simulink model "CAN_receiver"  (R2024a)
settings: Solver=FixedStepAuto  StartTime=0.0  StopTime=3  FixedStep=0.0025  RelTol=1e-3
undefined symbols (not defined in the file): CAN_Device, ImuSampleTime, Kvaser
libraries: sldrtlib x18
settings Model: Creator=17739  LastModifiedBy=17739
settings RTWCC: GPUComputeCapability=3.5

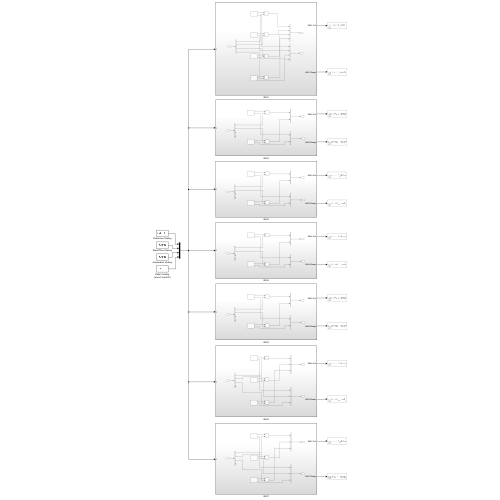
[thumbnail: Simulink's stored preview of the top-level diagram]
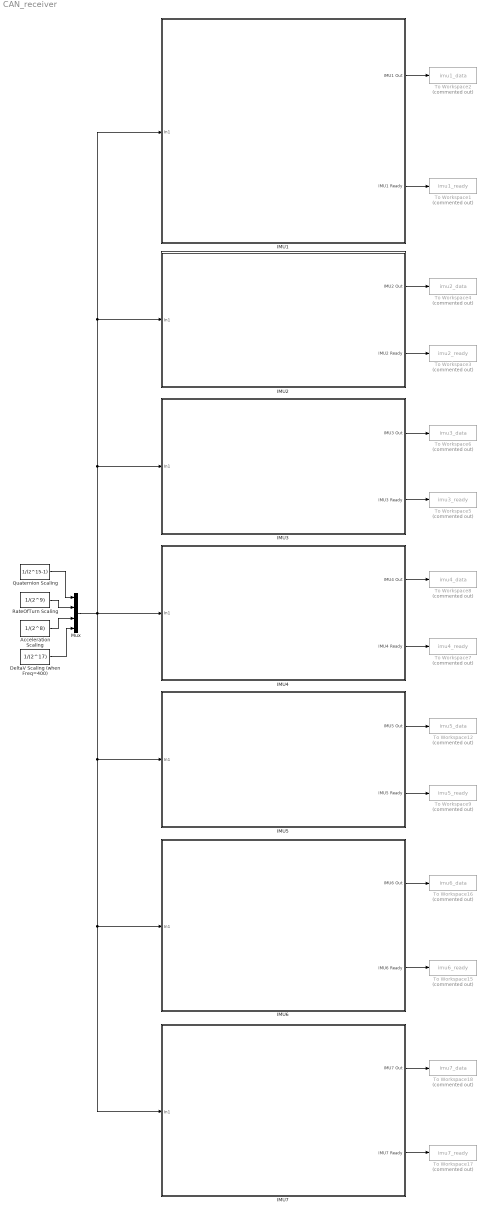
== system CAN_receiver ==
  Acceleration Scaling : Constant  Value=1/(2^8)
  DeltaV Scaling (when Freq=400) : Constant  Value=1/(2^17)
  IMU1 : Subsystem
  IMU2 : Subsystem
  IMU3 : Subsystem
  IMU4 : Subsystem
  IMU5 : Subsystem
  IMU6 : Subsystem
  IMU7 : Subsystem
  Mux : Mux
  Quaternion Scaling : Constant  Value=1/(2^15-1)
  RateOfTurn Scaling : Constant  Value=1/(2^9)
  To Workspace1 : ToWorkspace  Commented=on  VariableName=imu1_ready  SampleTime=-1
  To Workspace12 : ToWorkspace  Commented=on  VariableName=imu5_data  SampleTime=-1
  To Workspace15 : ToWorkspace  Commented=on  VariableName=imu6_ready  SampleTime=-1
  To Workspace16 : ToWorkspace  Commented=on  VariableName=imu6_data  SampleTime=-1
  To Workspace17 : ToWorkspace  Commented=on  VariableName=imu7_ready  SampleTime=-1
  To Workspace18 : ToWorkspace  Commented=on  VariableName=imu7_data  SampleTime=-1
  To Workspace2 : ToWorkspace  Commented=on  VariableName=imu1_data  SampleTime=-1
  To Workspace3 : ToWorkspace  Commented=on  VariableName=imu2_ready  SampleTime=-1
  To Workspace4 : ToWorkspace  Commented=on  VariableName=imu2_data  SampleTime=-1
  To Workspace5 : ToWorkspace  Commented=on  VariableName=imu3_ready  SampleTime=-1
  To Workspace6 : ToWorkspace  Commented=on  VariableName=imu3_data  SampleTime=-1
  To Workspace7 : ToWorkspace  Commented=on  VariableName=imu4_ready  SampleTime=-1
  To Workspace8 : ToWorkspace  Commented=on  VariableName=imu4_data  SampleTime=-1
  To Workspace9 : ToWorkspace  Commented=on  VariableName=imu5_ready  SampleTime=-1
  wires:
  IMU1/2(IMU1 Ready) -> To Workspace1/1
  IMU4/2(IMU4 Ready) -> To Workspace7/1
  RateOfTurn Scaling/1 -> Mux/2
  IMU7/2(IMU7 Ready) -> To Workspace17/1
  IMU5/2(IMU5 Ready) -> To Workspace9/1
  IMU3/2(IMU3 Ready) -> To Workspace5/1
  IMU2/2(IMU2 Ready) -> To Workspace3/1
  IMU3/1(IMU3 Out) -> To Workspace6/1
  IMU6/1(IMU6 Out) -> To Workspace16/1
  IMU4/1(IMU4 Out) -> To Workspace8/1
  DeltaV Scaling (when Freq=400)/1 -> Mux/4
  IMU5/1(IMU5 Out) -> To Workspace12/1
  IMU7/1(IMU7 Out) -> To Workspace18/1
  Quaternion Scaling/1 -> Mux/1
  IMU6/2(IMU6 Ready) -> To Workspace15/1
  Acceleration Scaling/1 -> Mux/3
  Mux/1 -> IMU7/1(In1), IMU6/1(In1), IMU5/1(In1), IMU4/1(In1), IMU3/1(In1), IMU1/1(In1), IMU2/1(In1)
  IMU2/1(IMU2 Out) -> To Workspace4/1
  IMU1/1(IMU1 Out) -> To Workspace2/1

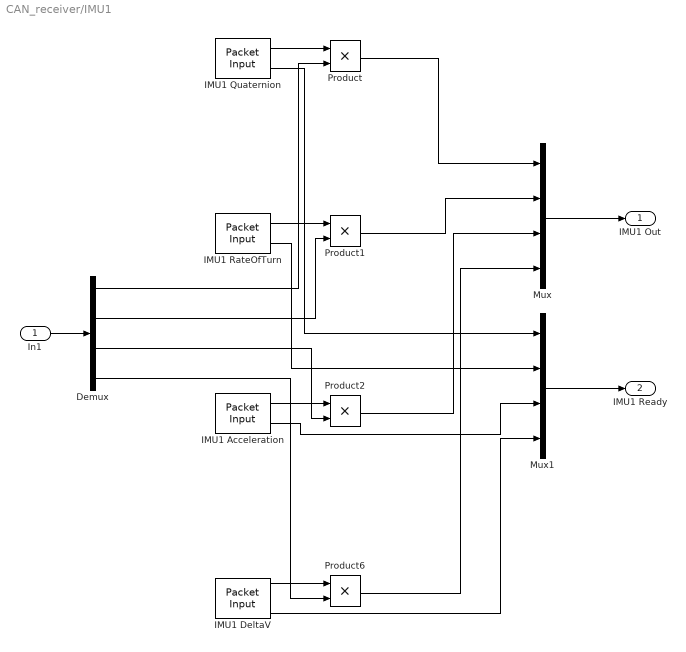
== system CAN_receiver/IMU1 ==
  In1 : Inport
  Demux : Demux
  IMU1 Acceleration : sldrtlib/Packet Input  SampleTime=ImuSampleTime  MaxMissedTicks=inf  ShowMissedTicks=off  YieldWhenWaiting=off  DrvName=Kvaser/CAN_Device  DrvAddress=0  DrvOptions=[0 0 0 0 1000 0 0]  PacketSize=6  DataTypes='3*int16'  ShowReady=on  ShowError=off  PacketID=2048e0 + (849)  ByteOrder=2  ShowTimestamp=off
      settings: AttributesFormatString=Kvaser\nCAN Device [0]
  IMU1 DeltaV : sldrtlib/Packet Input  SampleTime=ImuSampleTime  MaxMissedTicks=inf  ShowMissedTicks=off  YieldWhenWaiting=off  DrvName=Kvaser/CAN_Device  DrvAddress=0  DrvOptions=[0 0 0 0 1000 0 0]  PacketSize=7  DataTypes={'3*int16','uint8'}  ShowReady=on  ShowError=off  PacketID=2048e0 + (49)  ByteOrder=2  ShowTimestamp=off
      settings: AttributesFormatString=Kvaser\nCAN Device [0]
  IMU1 Quaternion : sldrtlib/Packet Input  SampleTime=ImuSampleTime  MaxMissedTicks=inf  ShowMissedTicks=off  YieldWhenWaiting=off  DrvName=Kvaser/CAN_Device  DrvAddress=0  DrvOptions=[0 0 0 0 1000 0 0]  PacketSize=8  DataTypes='4*int16'  ShowReady=on  ShowError=off  PacketID=2048e0 + (529)  ByteOrder=2  ShowTimestamp=off
      settings: AttributesFormatString=Kvaser\nCAN Device [0]
  IMU1 RateOfTurn : sldrtlib/Packet Input  SampleTime=ImuSampleTime  MaxMissedTicks=inf  ShowMissedTicks=off  YieldWhenWaiting=off  DrvName=Kvaser/CAN_Device  DrvAddress=0  DrvOptions=[0 0 0 0 1000 0 0]  PacketSize=6  DataTypes='3*int16'  ShowReady=on  ShowError=off  PacketID=2048e0 + (801)  ByteOrder=2  ShowTimestamp=off
      settings: AttributesFormatString=Kvaser\nCAN Device [0]
  Mux : Mux
  Mux1 : Mux
  Product{,1..2,6} (4 alike) : Product
  IMU1 Out : Outport
  IMU1 Ready : Outport  Port=2
  wires:
  Product/1 -> Mux/1
  Product1/1 -> Mux/2
  Product2/1 -> Mux/3
  Product6/1 -> Mux/4
  Mux/1 -> IMU1 Out/1
  In1/1 -> Demux/1
  IMU1 Quaternion/1 -> Product/1
  IMU1 RateOfTurn/1 -> Product1/1
  IMU1 Acceleration/1 -> Product2/1
  IMU1 DeltaV/1 -> Product6/1
  IMU1 Quaternion/2 -> Mux1/1
  IMU1 RateOfTurn/2 -> Mux1/2
  IMU1 Acceleration/2 -> Mux1/3
  IMU1 DeltaV/3 -> Mux1/4
  Demux/1 -> Product/2
  Demux/2 -> Product1/2
  Demux/3 -> Product2/2
  Demux/4 -> Product6/2
  Mux1/1 -> IMU1 Ready/1

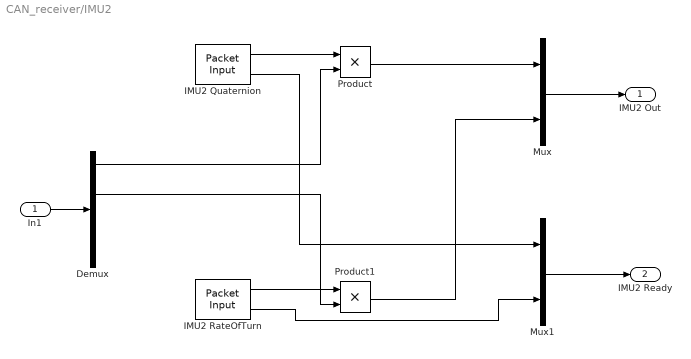
== system CAN_receiver/IMU2 ==
  In1 : Inport
  Demux : Demux
  IMU2 Quaternion : sldrtlib/Packet Input  SampleTime=ImuSampleTime  MaxMissedTicks=inf  ShowMissedTicks=off  YieldWhenWaiting=off  DrvName=Kvaser/CAN_Device  DrvAddress=0  DrvOptions=[0 0 0 0 1000 0 0]  PacketSize=8  DataTypes='4*int16'  ShowReady=on  ShowError=off  PacketID=2048e0 + (530)  ByteOrder=2  ShowTimestamp=off
      settings: AttributesFormatString=Kvaser\nCAN Device [0]
  IMU2 RateOfTurn : sldrtlib/Packet Input  SampleTime=ImuSampleTime  MaxMissedTicks=inf  ShowMissedTicks=off  YieldWhenWaiting=off  DrvName=Kvaser/CAN_Device  DrvAddress=0  DrvOptions=[0 0 0 0 1000 0 0]  PacketSize=6  DataTypes='3*int16'  ShowReady=on  ShowError=off  PacketID=2048e0 + (802)  ByteOrder=2  ShowTimestamp=off
      settings: AttributesFormatString=Kvaser\nCAN Device [0]
  Mux : Mux  Inputs=2
  Mux1 : Mux  Inputs=2
  Product : Product
  Product1 : Product
  IMU2 Out : Outport
  IMU2 Ready : Outport  Port=2
  wires:
  Mux/1 -> IMU2 Out/1
  In1/1 -> Demux/1
  Mux1/1 -> IMU2 Ready/1
  IMU2 RateOfTurn/1 -> Product1/1
  IMU2 Quaternion/1 -> Product/1
  Product/1 -> Mux/1
  Product1/1 -> Mux/2
  IMU2 RateOfTurn/2 -> Mux1/2
  IMU2 Quaternion/2 -> Mux1/1
  Demux/1 -> Product/2
  Demux/2 -> Product1/2

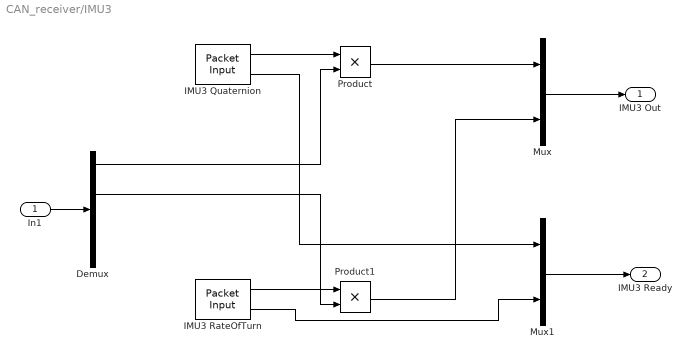
== system CAN_receiver/IMU3 ==
  In1 : Inport
  Demux : Demux
  IMU3 Quaternion : sldrtlib/Packet Input  SampleTime=ImuSampleTime  MaxMissedTicks=inf  ShowMissedTicks=off  YieldWhenWaiting=off  DrvName=Kvaser/CAN_Device  DrvAddress=0  DrvOptions=[0 0 0 0 1000 0 0]  PacketSize=8  DataTypes='4*int16'  ShowReady=on  ShowError=off  PacketID=2048e0 + (531)  ByteOrder=2  ShowTimestamp=off
      settings: AttributesFormatString=Kvaser\nCAN Device [0]
  IMU3 RateOfTurn : sldrtlib/Packet Input  SampleTime=ImuSampleTime  MaxMissedTicks=inf  ShowMissedTicks=off  YieldWhenWaiting=off  DrvName=Kvaser/CAN_Device  DrvAddress=0  DrvOptions=[0 0 0 0 1000 0 0]  PacketSize=6  DataTypes='3*int16'  ShowReady=on  ShowError=off  PacketID=2048e0 + (803)  ByteOrder=2  ShowTimestamp=off
      settings: AttributesFormatString=Kvaser\nCAN Device [0]
  Mux : Mux  Inputs=2
  Mux1 : Mux  Inputs=2
  Product : Product
  Product1 : Product
  IMU3 Out : Outport
  IMU3 Ready : Outport  Port=2
  wires:
  Mux/1 -> IMU3 Out/1
  In1/1 -> Demux/1
  Mux1/1 -> IMU3 Ready/1
  IMU3 RateOfTurn/1 -> Product1/1
  IMU3 Quaternion/1 -> Product/1
  Product/1 -> Mux/1
  Product1/1 -> Mux/2
  IMU3 RateOfTurn/2 -> Mux1/2
  IMU3 Quaternion/2 -> Mux1/1
  Demux/1 -> Product/2
  Demux/2 -> Product1/2

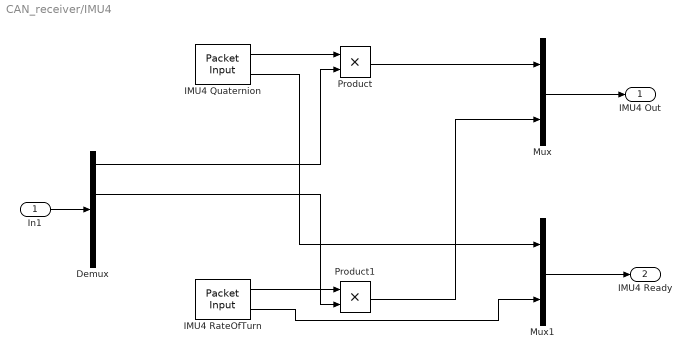
== system CAN_receiver/IMU4 ==
  In1 : Inport
  Demux : Demux
  IMU4 Quaternion : sldrtlib/Packet Input  SampleTime=ImuSampleTime  MaxMissedTicks=inf  ShowMissedTicks=off  YieldWhenWaiting=off  DrvName=Kvaser/CAN_Device  DrvAddress=0  DrvOptions=[0 0 0 0 1000 0 0]  PacketSize=8  DataTypes='4*int16'  ShowReady=on  ShowError=off  PacketID=2048e0 + (532)  ByteOrder=2  ShowTimestamp=off
      settings: AttributesFormatString=Kvaser\nCAN Device [0]
  IMU4 RateOfTurn : sldrtlib/Packet Input  SampleTime=ImuSampleTime  MaxMissedTicks=inf  ShowMissedTicks=off  YieldWhenWaiting=off  DrvName=Kvaser/CAN_Device  DrvAddress=0  DrvOptions=[0 0 0 0 1000 0 0]  PacketSize=6  DataTypes='3*int16'  ShowReady=on  ShowError=off  PacketID=2048e0 + (804)  ByteOrder=2  ShowTimestamp=off
      settings: AttributesFormatString=Kvaser\nCAN Device [0]
  Mux : Mux  Inputs=2
  Mux1 : Mux  Inputs=2
  Product : Product
  Product1 : Product
  IMU4 Out : Outport
  IMU4 Ready : Outport  Port=2
  wires:
  Mux/1 -> IMU4 Out/1
  In1/1 -> Demux/1
  Mux1/1 -> IMU4 Ready/1
  IMU4 RateOfTurn/1 -> Product1/1
  IMU4 Quaternion/1 -> Product/1
  Product/1 -> Mux/1
  Product1/1 -> Mux/2
  IMU4 RateOfTurn/2 -> Mux1/2
  IMU4 Quaternion/2 -> Mux1/1
  Demux/1 -> Product/2
  Demux/2 -> Product1/2

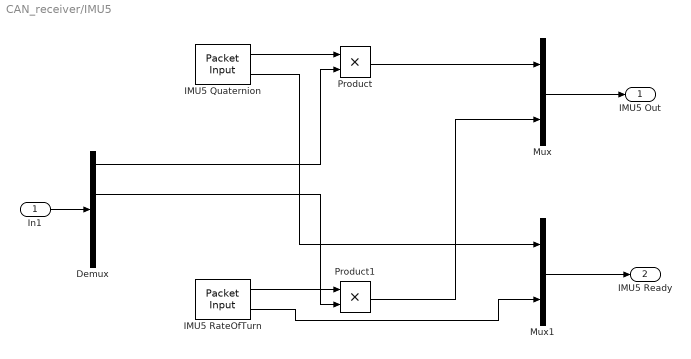
== system CAN_receiver/IMU5 ==
  In1 : Inport
  Demux : Demux
  IMU5 Quaternion : sldrtlib/Packet Input  SampleTime=ImuSampleTime  MaxMissedTicks=inf  ShowMissedTicks=off  YieldWhenWaiting=off  DrvName=Kvaser/CAN_Device  DrvAddress=0  DrvOptions=[0 0 0 0 1000 0 0]  PacketSize=8  DataTypes='4*int16'  ShowReady=on  ShowError=off  PacketID=2048e0 + (533)  ByteOrder=2  ShowTimestamp=off
      settings: AttributesFormatString=Kvaser\nCAN Device [0]
  IMU5 RateOfTurn : sldrtlib/Packet Input  SampleTime=ImuSampleTime  MaxMissedTicks=inf  ShowMissedTicks=off  YieldWhenWaiting=off  DrvName=Kvaser/CAN_Device  DrvAddress=0  DrvOptions=[0 0 0 0 1000 0 0]  PacketSize=6  DataTypes='3*int16'  ShowReady=on  ShowError=off  PacketID=2048e0 + (805)  ByteOrder=2  ShowTimestamp=off
      settings: AttributesFormatString=Kvaser\nCAN Device [0]
  Mux : Mux  Inputs=2
  Mux1 : Mux  Inputs=2
  Product : Product
  Product1 : Product
  IMU5 Out : Outport
  IMU5 Ready : Outport  Port=2
  wires:
  Mux/1 -> IMU5 Out/1
  In1/1 -> Demux/1
  Mux1/1 -> IMU5 Ready/1
  IMU5 RateOfTurn/1 -> Product1/1
  IMU5 Quaternion/1 -> Product/1
  Product/1 -> Mux/1
  Product1/1 -> Mux/2
  IMU5 RateOfTurn/2 -> Mux1/2
  IMU5 Quaternion/2 -> Mux1/1
  Demux/1 -> Product/2
  Demux/2 -> Product1/2

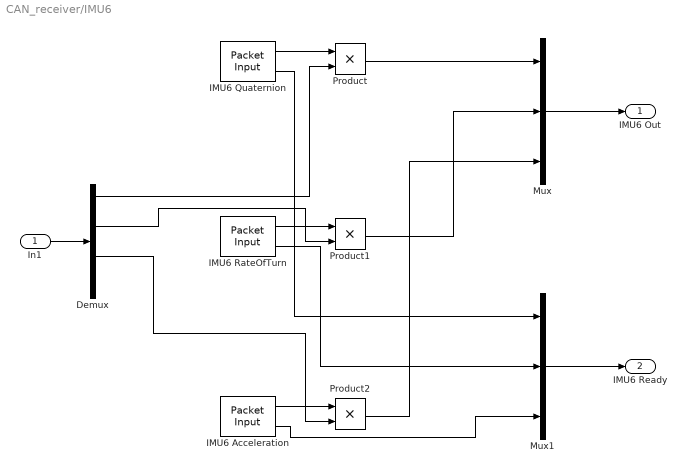
== system CAN_receiver/IMU6 ==
  In1 : Inport
  Demux : Demux
  IMU6 Acceleration : sldrtlib/Packet Input  SampleTime=ImuSampleTime  MaxMissedTicks=inf  ShowMissedTicks=off  YieldWhenWaiting=off  DrvName=Kvaser/CAN_Device  DrvAddress=0  DrvOptions=[0 0 0 0 1000 0 0]  PacketSize=6  DataTypes='3*int16'  ShowReady=on  ShowError=off  PacketID=2048e0 + (854)  ByteOrder=2  ShowTimestamp=off
      settings: AttributesFormatString=Kvaser\nCAN Device [0]
  IMU6 Quaternion : sldrtlib/Packet Input  SampleTime=ImuSampleTime  MaxMissedTicks=inf  ShowMissedTicks=off  YieldWhenWaiting=off  DrvName=Kvaser/CAN_Device  DrvAddress=0  DrvOptions=[0 0 0 0 1000 0 0]  PacketSize=8  DataTypes='4*int16'  ShowReady=on  ShowError=off  PacketID=2048e0 + (534)  ByteOrder=2  ShowTimestamp=off
      settings: AttributesFormatString=Kvaser\nCAN Device [0]
  IMU6 RateOfTurn : sldrtlib/Packet Input  SampleTime=ImuSampleTime  MaxMissedTicks=inf  ShowMissedTicks=off  YieldWhenWaiting=off  DrvName=Kvaser/CAN_Device  DrvAddress=0  DrvOptions=[0 0 0 0 1000 0 0]  PacketSize=6  DataTypes='3*int16'  ShowReady=on  ShowError=off  PacketID=2048e0 + (806)  ByteOrder=2  ShowTimestamp=off
      settings: AttributesFormatString=Kvaser\nCAN Device [0]
  Mux : Mux  Inputs=3
  Mux1 : Mux  Inputs=3
  Product : Product
  Product1 : Product
  Product2 : Product
  IMU6 Out : Outport
  IMU6 Ready : Outport  Port=2
  wires:
  Mux/1 -> IMU6 Out/1
  In1/1 -> Demux/1
  IMU6 Quaternion/1 -> Product/1
  IMU6 RateOfTurn/1 -> Product1/1
  IMU6 Acceleration/1 -> Product2/1
  Mux1/1 -> IMU6 Ready/1
  Demux/1 -> Product/2
  Demux/2 -> Product1/2
  Demux/3 -> Product2/2
  Product/1 -> Mux/1
  Product1/1 -> Mux/2
  Product2/1 -> Mux/3
  IMU6 Quaternion/2 -> Mux1/1
  IMU6 RateOfTurn/2 -> Mux1/2
  IMU6 Acceleration/2 -> Mux1/3

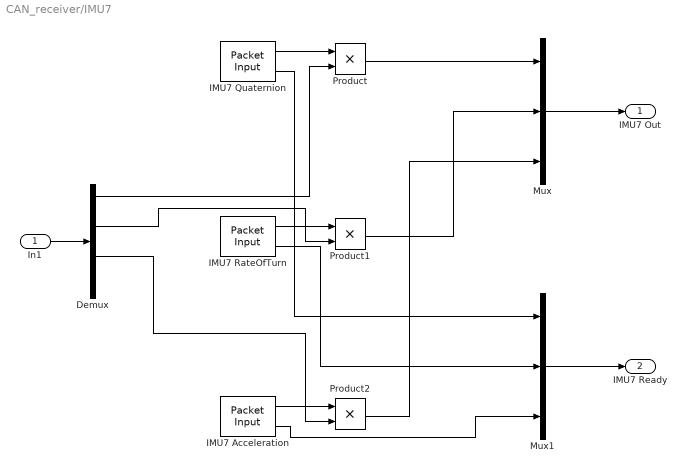
== system CAN_receiver/IMU7 ==
  In1 : Inport
  Demux : Demux
  IMU7 Acceleration : sldrtlib/Packet Input  SampleTime=ImuSampleTime  MaxMissedTicks=inf  ShowMissedTicks=off  YieldWhenWaiting=off  DrvName=Kvaser/CAN_Device  DrvAddress=0  DrvOptions=[0 0 0 0 1000 0 0]  PacketSize=6  DataTypes='3*int16'  ShowReady=on  ShowError=off  PacketID=2048e0 + (855)  ByteOrder=2  ShowTimestamp=off
      settings: AttributesFormatString=Kvaser\nCAN Device [0]
  IMU7 Quaternion : sldrtlib/Packet Input  SampleTime=ImuSampleTime  MaxMissedTicks=inf  ShowMissedTicks=off  YieldWhenWaiting=off  DrvName=Kvaser/CAN_Device  DrvAddress=0  DrvOptions=[0 0 0 0 1000 0 0]  PacketSize=8  DataTypes='4*int16'  ShowReady=on  ShowError=off  PacketID=2048e0 + (535)  ByteOrder=2  ShowTimestamp=off
      settings: AttributesFormatString=Kvaser\nCAN Device [0]
  IMU7 RateOfTurn : sldrtlib/Packet Input  SampleTime=ImuSampleTime  MaxMissedTicks=inf  ShowMissedTicks=off  YieldWhenWaiting=off  DrvName=Kvaser/CAN_Device  DrvAddress=0  DrvOptions=[0 0 0 0 1000 0 0]  PacketSize=6  DataTypes='3*int16'  ShowReady=on  ShowError=off  PacketID=2048e0 + (807)  ByteOrder=2  ShowTimestamp=off
      settings: AttributesFormatString=Kvaser\nCAN Device [0]
  Mux : Mux  Inputs=3
  Mux1 : Mux  Inputs=3
  Product : Product
  Product1 : Product
  Product2 : Product
  IMU7 Out : Outport
  IMU7 Ready : Outport  Port=2
  wires:
  Mux/1 -> IMU7 Out/1
  In1/1 -> Demux/1
  IMU7 Quaternion/1 -> Product/1
  IMU7 RateOfTurn/1 -> Product1/1
  IMU7 Acceleration/1 -> Product2/1
  Mux1/1 -> IMU7 Ready/1
  Demux/1 -> Product/2
  Demux/2 -> Product1/2
  Demux/3 -> Product2/2
  Product/1 -> Mux/1
  Product1/1 -> Mux/2
  Product2/1 -> Mux/3
  IMU7 Quaternion/2 -> Mux1/1
  IMU7 RateOfTurn/2 -> Mux1/2
  IMU7 Acceleration/2 -> Mux1/3
